simulink model "verify_Pump_Const_mdl"  (R2016b)
settings: Solver=ode45  StartTime=0.0  StopTime=240  MaxStep=1  RelTol=1e-3  EnableMultiTasking=on
libraries: carnot x2
settings Model: Creator=drhf  LastModifiedBy=srrt
settings DataIOCC: SaveFormat=Array  SignalLoggingSaveFormat=ModelDataLogs
settings OptimizationCC: ExpressionDepthLimit=2147483647  LifeSpan=inf
settings DebuggingCC: UnderspecifiedInitializationDetection=Classic  MergeDetectMultiDrivingBlocksExec=none  SolverPrmCheckMsg=warning  FcnCallInpInsideContextMsg=warning  StateNameClashWarn=warning  SFUnexpectedBacktrackingDiag=warning  SFNoUnconditionalDefaultTransitionDiag=warning  SFExecutionAtInitializationDiag=none
settings HardwareCC: ProdBitPerPointer=32  ProdBitPerSizeT=32  ProdBitPerPtrDiffT=32  ProdLargestAtomicFloat=None  ProdIntDivRoundTo=Undefined  ProdEndianess=Unspecified  ProdWordSize=32  ProdHWDeviceType=32-bit Generic
settings ModelReferenceCC: PropagateSignalLabelsOutOfModel=off
settings GRTTargetCC: TargetLangStandard=C89/C90 (ANSI)  GeneratePreprocessorConditionals=Disable all  CombineOutputUpdateFcns=off  GRTInterface=on
settings ConfigComp: CovMetricSettings=dw  CovHtmlReporting=on  CovSaveCumulativeToWorkspaceVar=on  CovSaveSingleToWorkspaceVar=on  CovExternalEMLEnable=off

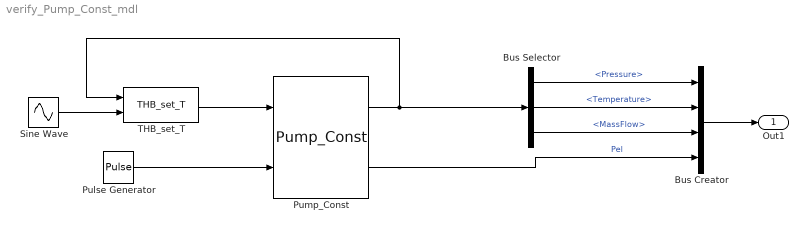
== system verify_Pump_Const_mdl ==
  Bus Creator : BusCreator  Inputs=4
  Bus Selector : BusSelector  OutputSignals=Pressure,Temperature,MassFlow
  Pulse Generator : DiscretePulseGenerator  PulseType=Time based  Period=120  PulseWidth=50
  Pump_Const : carnot/Hydraulics/Pump_Const  mdotmax=1200/3600  dia=0.0157  power=30  p0=3e5  fluid_id=Water  mix=0  UA=3  mcp=4000  tamb=20
  Sine Wave : Sin  Amplitude=5  Bias=20  Frequency=2*pi/240  SampleTime=0
  THB_set_T : carnot/Source/Simple/THB_set_T
  Out1 : Outport
  wires:
  Bus Creator/1 -> Out1/1
  Bus Selector/3 -> Bus Creator/3  "<MassFlow>"
  Pulse Generator/1 -> Pump_Const/2
  Pump_Const/1 -> THB_set_T/1, Bus Selector/1
  Pump_Const/2 -> Bus Creator/4  "Pel"
  Bus Selector/1 -> Bus Creator/1  "<Pressure>"
  Bus Selector/2 -> Bus Creator/2  "<Temperature>"
  Sine Wave/1 -> THB_set_T/2
  THB_set_T/1 -> Pump_Const/1
